simulink model "turbine_generator_model"  (R2024a)
settings: Solver=ode45  StartTime=0.0  StopTime=15  RelTol=1e-3
undefined symbols (not defined in the file): J
settings Model: Creator=MUSU  LastModifiedBy=MUSU

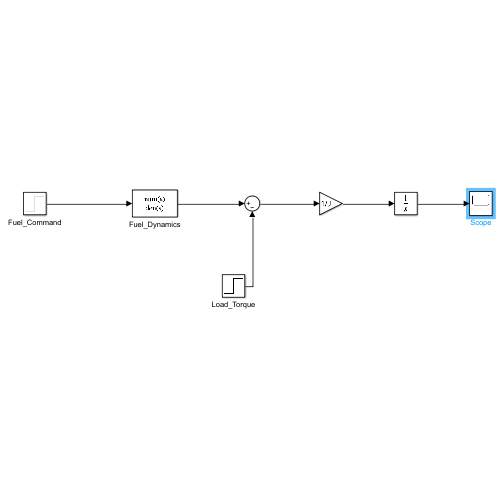
[thumbnail: Simulink's stored preview of the top-level diagram]
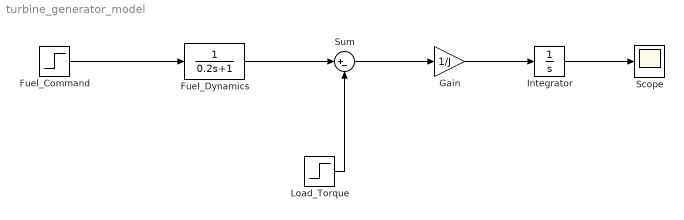
== system turbine_generator_model ==
  Fuel_Command : Step  Time=0  SampleTime=0
  Fuel_Dynamics : TransferFcn  Denominator=[0.2 1]
  Gain : Gain  Gain=1/J
  Integrator : Integrator
  Load_Torque : Step  Time=5  After=0.7  SampleTime=0
  Scope : Scope
  Sum : Sum  Inputs=|+-
  wires:
  Fuel_Command/1 -> Fuel_Dynamics/1
  Fuel_Dynamics/1 -> Sum/1
  Sum/1 -> Gain/1
  Gain/1 -> Integrator/1
  Integrator/1 -> Scope/1
  Load_Torque/1 -> Sum/2
